simulink model "ALFC_vinay"  (R2017a)
settings: Solver=VariableStepAuto  StartTime=0.0  StopTime=20  FixedStep=0.01  MaxStep=1e-4  RelTol=1e-3
libraries: simulink x1, powerlib x1
settings Model: Creator=HP  LastModifiedBy=HP

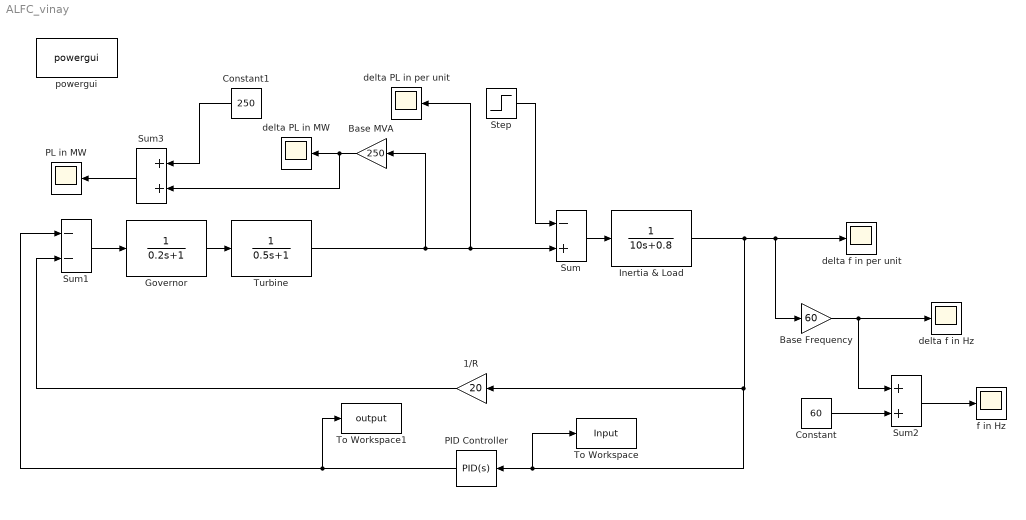
== system ALFC_vinay ==
  1/R : Gain  Gain=20
  Base Frequency : Gain  Gain=60
  Base MVA : Gain  Gain=250
  Constant : Constant  Value=60
  Constant1 : Constant  Value=250
  Governor : TransferFcn  Denominator=[0.2 1]
  Inertia & Load : TransferFcn  Denominator=[10 0.8]
  PID Controller : simulink/Continuous/PID Controller  Controller=PID  TimeDomain=Continuous-time  SampleTime=-1  IntegratorMethod=Forward Euler  FilterMethod=Forward Euler  Form=Parallel  UseFilter=on  ControllerParametersSource=internal  P=50  I=30  D=10  N=100  InitialConditionSource=internal  InitialConditionForIntegrator=0  InitialConditionForFilter=0  ExternalReset=none  LimitOutput=off  UpperSaturationLimit=inf  LowerSaturationLimit=-inf  LinearizeAsGain=on  AntiWindupMode=none  Kb=1  TrackingMode=off  Kt=1  PParamMin=[]  PParamMax=[]  IParamMin=[]  IParamMax=[]  DParamMin=[]  DParamMax=[]  NParamMin=[]  NParamMax=[]  KbParamMin=[]  KbParamMax=[]  KtParamMin=[]  KtParamMax=[]  POutMin=[]  POutMax=[]  IOutMin=[]  IOutMax=[]  DOutMin=[]  DOutMax=[]  NOutMin=[]  NOutMax=[]  KbOutMin=[]  KbOutMax=[]  KtOutMin=[]  KtOutMax=[]  IntegratorOutMin=[]  IntegratorOutMax=[]  FilterOutMin=[]  FilterOutMax=[]  SumOutMin=[]  SumOutMax=[]  SumI1OutMin=[]  SumI1OutMax=[]  SumI2OutMin=[]  SumI2OutMax=[]  SumI3OutMin=[]  SumI3OutMax=[]  SumDOutMin=[]  SumDOutMax=[]  SaturationOutMin=[]  SaturationOutMax=[]  IntegratorContinuousStateAttributes=''  IntegratorStateMustResolveToSignalObject=off  IntegratorRTWStateStorageClass=Auto  FilterContinuousStateAttributes=''  FilterStateMustResolveToSignalObject=off  FilterRTWStateStorageClass=Auto  DifferentiatorICPrevScaledInput=0  DifferentiatorOutMin=[]  DifferentiatorOutMax=[]  InitialConditionSetting=State (most efficient)
  PL in MW : Scope
  Step : Step  Time=100  Before=0.2  After=0.2  SampleTime=0
  Sum : Sum  Inputs=-+
  Sum1 : Sum  Inputs=--
  Sum2 : Sum
  Sum3 : Sum
  To Workspace : ToWorkspace  VariableName=Input  SampleTime=-1
  To Workspace1 : ToWorkspace  VariableName=output  SampleTime=-1
  Turbine : TransferFcn  Denominator=[0.5 1]
  delta PL in MW : Scope
  delta PL in per unit : Scope
  delta f in Hz : Scope
  delta f in per unit : Scope
  f in Hz : Scope
  powergui : powerlib/powergui  Priority=1  SimulationMode=Continuous  SampleTime=0.01  frequency=60  Iterations=50  frequencyindice=60  Pbase=100e6  ErrMax=1e-4  UnitsV=kV  UnitsW=MW  buscounter=0  FunctionMessages=off  echomessages=off  EnableUseOfTLC=off  CurrentSourceSwitches=off  DisableSnubberDevices=off  DisableRonSwitches=off  DisableVfSwitches=off  DisplayEquations=off  SolverType=Tustin/Backward Euler (TBE)  Interpol=off  ExternalGateDelay=off  methode=off  Ts=100  x0status=blocks  SPID=on  SwTol=0  HookPort=off  RestoreLinks=warning  ResistiveCurrentMeasurement=off  Frange=[0:2:500]  Ylog=off  Xlog=on  ShowGrid=off  save=off  variable=ZData  structure=0  ZoomFFT=off  StartTime=0.0  cycles=1  DisplayStyle=1  fundamental=60  FreqAxis=off  MaxFrequency=1000  frequencyindicesteady=1  RmsSteady=1  display=off
  wires:
  Governor/1 -> Turbine/1
  Turbine/1 -> Base MVA/1, delta PL in per unit/1, Sum/2
  Step/1 -> Sum/1
  Sum/1 -> Inertia & Load/1
  Inertia & Load/1 -> Base Frequency/1, delta f in per unit/1, To Workspace/1, PID Controller/1, 1/R/1
  Sum1/1 -> Governor/1
  Base Frequency/1 -> Sum2/1, delta f in Hz/1
  Constant/1 -> Sum2/2
  Sum2/1 -> f in Hz/1
  Base MVA/1 -> Sum3/2, delta PL in MW/1
  Constant1/1 -> Sum3/1
  Sum3/1 -> PL in MW/1
  1/R/1 -> Sum1/2
  PID Controller/1 -> To Workspace1/1, Sum1/1
